simulink model "HW3_sim"  (R2024b)
settings: Solver=VariableStepAuto  StartTime=0.0  StopTime=sim_time  FixedStep=1  RelTol=1e-8  AbsTol=1e-8
values from neighbouring files (symbols this model uses):
  Ag0 = [sind(theta) 0 -sind(theta) 0; 0 sind(theta) 0 -sind(theta); cosd(theta) cosd(theta) cosd(theta) cosd(theta)]    [CMG_init_script.m]    (also in HW3_init_script.m)
  As0 = [sind(theta) 0 -sind(theta) 0; 0 sind(theta) 0 -sind(theta); cosd(theta) cosd(theta) cosd(theta) cosd(theta)]    [HW3_init_script.m]
  At0 = [-cosd(theta) 0 cosd(theta) 0; 0 -cosd(theta) 0 cosd(theta); sind(theta) sind(theta) sind(theta) sind(theta)]    [CMG_init_script.m]    (also in HW3_init_script.m)
  CMG = boolean(1)    [CMG_init_script.m]    (also in HW3_init_script.m)
  E0_body_ECI = euler_from_C(C0_body_ECI)    [CMG_init_script.m]    (also in HW3_init_script.m)
  E0_body_LVLH = euler_from_C(C0_body_LVLH)    [CMG_init_script.m]    (also in HW3_init_script.m)
  gamma0 = [0;0;0;0]    [CMG_init_script.m]    (also in HW3_init_script.m)
  I_b = 1/12*m_sc*diag([y^2 + z^2; x^2 + z^2; x^2 + y^2])    [CMG_init_script.m]    (also in HW3_init_script.m)
  I_cg = [I_CMG1(1,1) 0 0 0; 0 I_CMG2(1,1) 0 0; 0 0 I_CMG3(1,1) 0; 0 0 0 I_CMG4(1,1)]    [CMG_init_script.m]    (also in HW3_init_script.m)
  I_cs = I_ws    [CMG_init_script.m]    (also in HW3_init_script.m)
  I_ct = [I_CMG1(2,2) 0 0 0; 0 I_CMG2(2,2) 0 0; 0 0 I_CMG3(2,2) 0; 0 0 0 I_CMG4(2,2)]    [CMG_init_script.m]    (also in HW3_init_script.m)
  I_ws = [I_CMG1(3,3) 0 0 0; 0 I_CMG2(3,3) 0 0; 0 0 I_CMG3(3,3) 0; 0 0 0 I_CMG4(3,3)]    [CMG_init_script.m]    (also in HW3_init_script.m)
  J_sc = I_b + As0*I_cs*As0' + At0*I_ct*At0' + Ag0*I_cg*Ag0'    [CMG_init_script.m]    (also in HW3_init_script.m)
  K_d = 2*zeta*omega_n*J_sc    [CMG_init_script.m]    (also in HW3_init_script.m)
  K_p = 2*omega_n^2 * J_sc    [CMG_init_script.m]    (also in HW3_init_script.m)
  n_sc = (2*pi)/period    [CMG_init_script.m]    (also in HW3_init_script.m)
  Omega0 = [800; 800; 800; 800]    [CMG_init_script.m]    (also in HW3_init_script.m)
  omega0_body_ECI = 10^-3 * [0.5; -0.2; -3]    [CMG_init_script.m]    (also in HW3_init_script.m)
  q0_body_ECI = [0.5; 0.5; 0.5; 0.5]    [CMG_init_script.m]    (also in HW3_init_script.m)
  q0_body_LVLH = C2quat(C0_body_LVLH)    [CMG_init_script.m]    (also in HW3_init_script.m)
  q_c = [0; 0; 0; 1]    [CMG_init_script.m]    (also in HW3_init_script.m)
  r0 = r0'    [CMG_init_script.m]    (also in HW3_init_script.m)
  RW = boolean(0)    [CMG_init_script.m]    (also in HW3_init_script.m)
  T_d0 = 10^-5 * [0; 0.5; 0]    [CMG_init_script.m]    (also in HW3_init_script.m)
  v0 = v0'    [CMG_init_script.m]    (also in HW3_init_script.m)
settings Model: Creator=josep  LastModifiedBy=josep
settings DataIOCC: SaveFormat=StructureWithTime

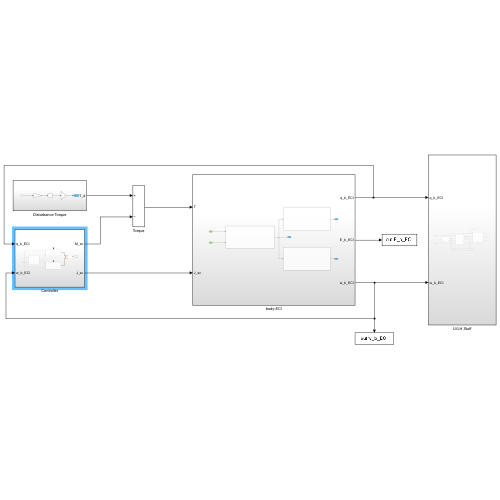
[thumbnail: Simulink's stored preview of the top-level diagram]
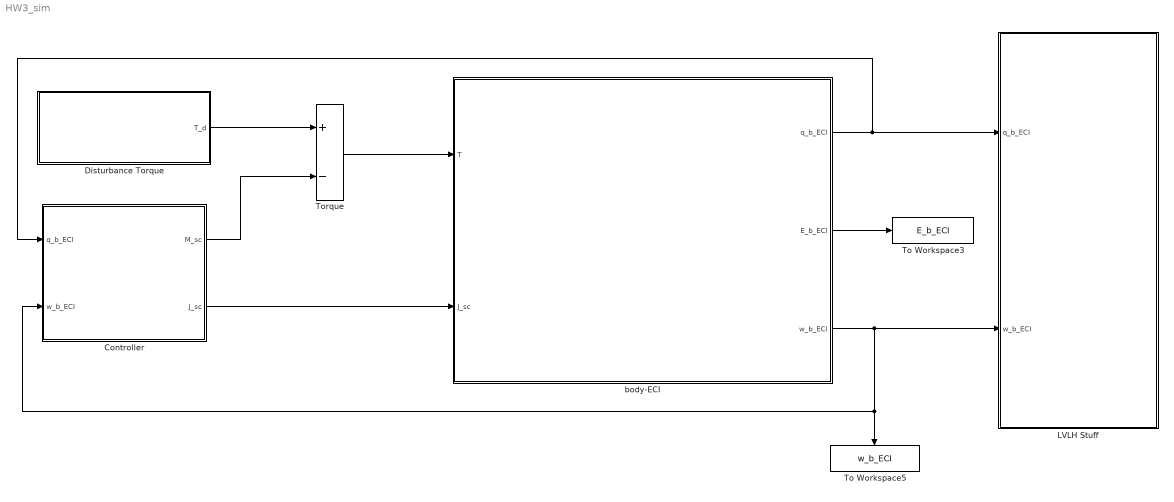
== system HW3_sim ==
  Controller : Subsystem
  Disturbance Torque : Subsystem
  LVLH Stuff : Subsystem
  To Workspace3 : ToWorkspace  VariableName=E_b_ECI  SampleTime=-1
  To Workspace5 : ToWorkspace  VariableName=w_b_ECI  SampleTime=-1
  Torque : Sum  Inputs=+-
  body-ECI : Subsystem
  wires:
  body-ECI/3(w_b_ECI) -> To Workspace5/1, Controller/2(w_b_ECI), LVLH Stuff/2(w_b_ECI)
  body-ECI/2(E_b_ECI) -> To Workspace3/1
  Torque/1 -> body-ECI/1(T)
  body-ECI/1(q_b_ECI) -> Controller/1(q_b_ECI), LVLH Stuff/1(q_b_ECI)
  Disturbance Torque/1(T_d) -> Torque/1
  Controller/2(J_sc) -> body-ECI/2(J_sc)
  Controller/1(M_sc) -> Torque/2

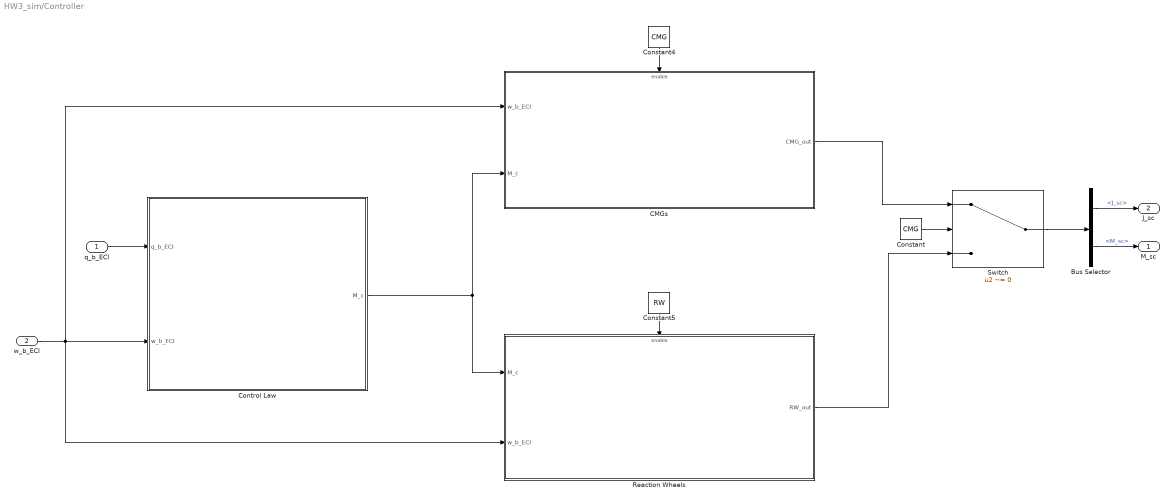
== system HW3_sim/Controller ==
  q_b_ECI : Inport
  w_b_ECI : Inport  Port=2
  Bus Selector : BusSelector  OutputSignals=J_sc,M_sc
  CMGs : Subsystem
  Constant : Constant  Value=CMG
  Constant4 : Constant  Value=CMG
  Constant5 : Constant  Value=RW
  Control Law : Subsystem
  Reaction Wheels : Subsystem
  Switch : Switch  Criteria=u2 ~= 0  SaturateOnIntegerOverflow=off  InputSameDT=off
  M_sc : Outport
  J_sc : Outport  Port=2
  wires:
  w_b_ECI/1 -> Reaction Wheels/2(w_b_ECI), CMGs/1(w_b_ECI), Control Law/2(w_b_ECI)
  Constant/1 -> Switch/2
  Constant4/1 -> CMGs/Enable
  Constant5/1 -> Reaction Wheels/Enable
  Switch/1 -> Bus Selector/1
  Bus Selector/1 -> J_sc/1  "<J_sc>"
  Bus Selector/2 -> M_sc/1  "<M_sc>"
  Control Law/1(M_c) -> CMGs/2(M_c), Reaction Wheels/1(M_c)
  q_b_ECI/1 -> Control Law/1(q_b_ECI)
  CMGs/1(CMG_out) -> Switch/1
  Reaction Wheels/1(RW_out) -> Switch/3

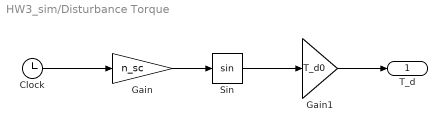
== system HW3_sim/Disturbance Torque ==
  Clock : Clock
  Gain : Gain  Gain=n_sc
  Gain1 : Gain  Gain=T_d0
  Sin : Trigonometry
  T_d : Outport
  wires:
  Gain1/1 -> T_d/1
  Clock/1 -> Gain/1
  Gain/1 -> Sin/1
  Sin/1 -> Gain1/1

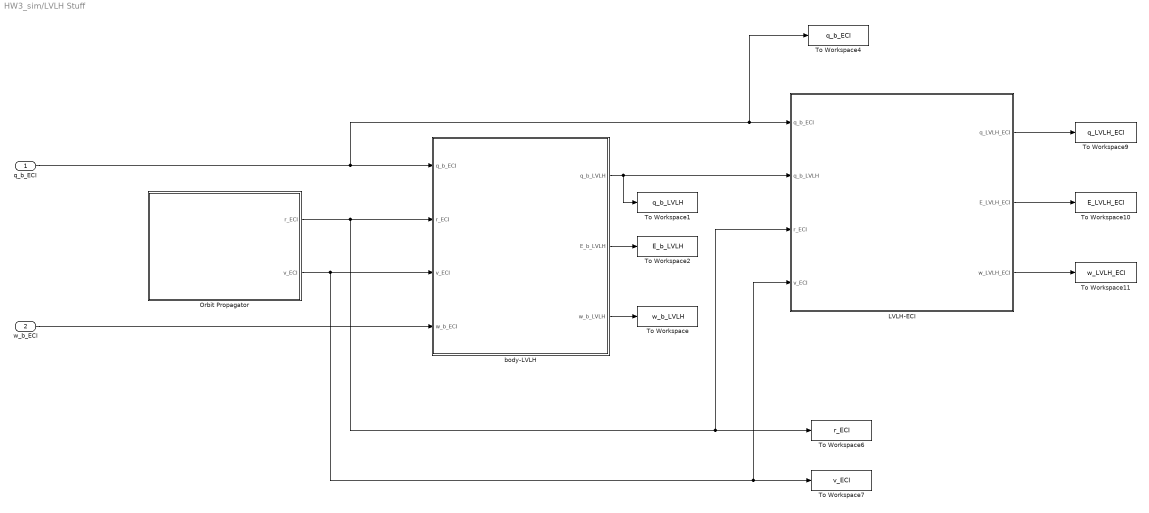
== system HW3_sim/LVLH Stuff ==
  q_b_ECI : Inport
  w_b_ECI : Inport  Port=2
  LVLH-ECI : Subsystem
  Orbit Propagator : Subsystem
  To Workspace : ToWorkspace  VariableName=w_b_LVLH  SampleTime=-1
  To Workspace1 : ToWorkspace  VariableName=q_b_LVLH  SampleTime=-1
      settings: Save2DSignal=2-D array (concatenate along first dimension)
  To Workspace10 : ToWorkspace  VariableName=E_LVLH_ECI  SampleTime=-1
  To Workspace11 : ToWorkspace  VariableName=w_LVLH_ECI  SampleTime=-1
  To Workspace2 : ToWorkspace  VariableName=E_b_LVLH  SampleTime=-1
  To Workspace4 : ToWorkspace  VariableName=q_b_ECI  SampleTime=-1
  To Workspace6 : ToWorkspace  VariableName=r_ECI  SampleTime=-1
  To Workspace7 : ToWorkspace  VariableName=v_ECI  SampleTime=-1
  To Workspace9 : ToWorkspace  VariableName=q_LVLH_ECI  SampleTime=-1
  body-LVLH : Subsystem
  wires:
  q_b_ECI/1 -> LVLH-ECI/1(q_b_ECI), To Workspace4/1, body-LVLH/1(q_b_ECI)
  body-LVLH/3(w_b_LVLH) -> To Workspace/1
  Orbit Propagator/2(v_ECI) -> body-LVLH/3(v_ECI), LVLH-ECI/4(v_ECI), To Workspace7/1
  body-LVLH/2(E_b_LVLH) -> To Workspace2/1
  LVLH-ECI/1(q_LVLH_ECI) -> To Workspace9/1
  Orbit Propagator/1(r_ECI) -> body-LVLH/2(r_ECI), To Workspace6/1, LVLH-ECI/3(r_ECI)
  LVLH-ECI/3(w_LVLH_ECI) -> To Workspace11/1
  body-LVLH/1(q_b_LVLH) -> LVLH-ECI/2(q_b_LVLH), To Workspace1/1
  LVLH-ECI/2(E_LVLH_ECI) -> To Workspace10/1
  w_b_ECI/1 -> body-LVLH/4(w_b_ECI)

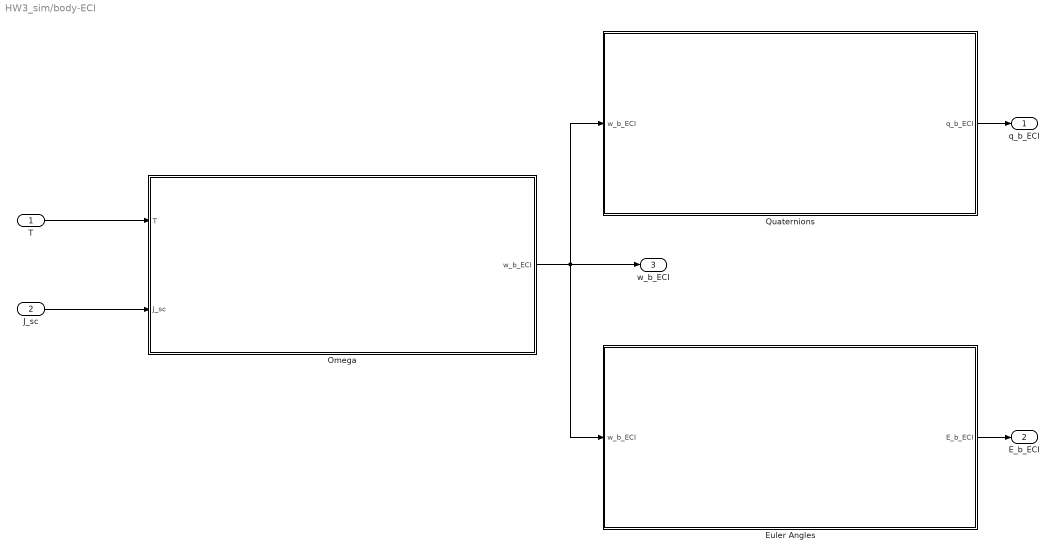
== system HW3_sim/body-ECI ==
  T : Inport
  J_sc : Inport  Port=2
  Euler Angles : Subsystem
  Omega : Subsystem
  Quaternions : Subsystem
  q_b_ECI : Outport
  E_b_ECI : Outport  Port=2
  w_b_ECI : Outport  Port=3
  wires:
  Omega/1(w_b_ECI) -> Quaternions/1(w_b_ECI), Euler Angles/1(w_b_ECI), w_b_ECI/1
  Euler Angles/1(E_b_ECI) -> E_b_ECI/1
  Quaternions/1(q_b_ECI) -> q_b_ECI/1
  T/1 -> Omega/1(T)
  J_sc/1 -> Omega/2(J_sc)

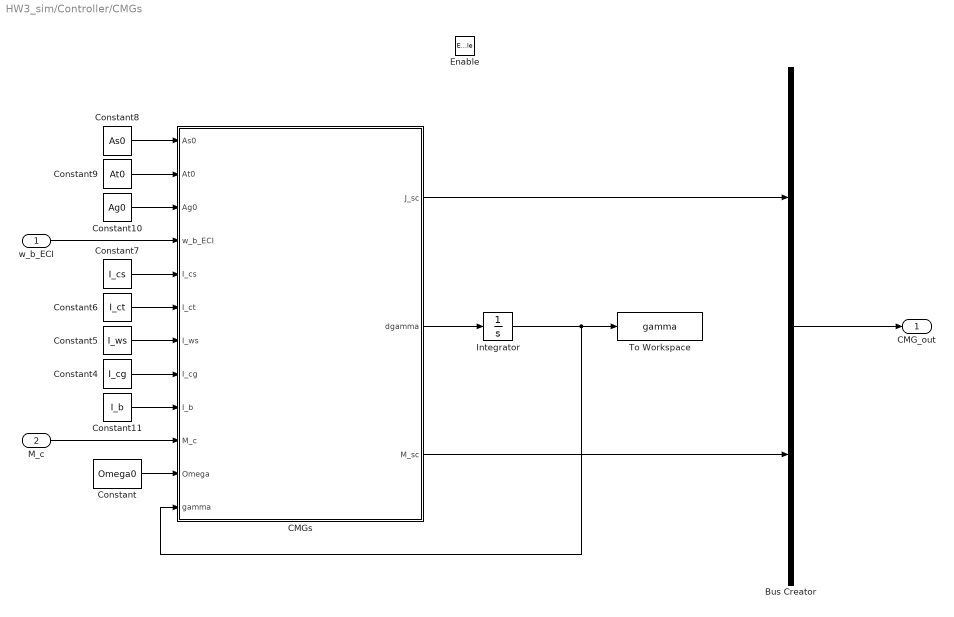
== system HW3_sim/Controller/CMGs ==
  w_b_ECI : Inport
  M_c : Inport  Port=2
  Enable : EnablePort
  Bus Creator : BusCreator  Inputs=2
  CMGs : MATLAB Function  TreatAsAtomicUnit=on
  Constant : Constant  Value=Omega0
  Constant10 : Constant  Value=Ag0
  Constant11 : Constant  Value=I_b
  Constant4 : Constant  Value=I_cg
  Constant5 : Constant  Value=I_ws
  Constant6 : Constant  Value=I_ct
  Constant7 : Constant  Value=I_cs
  Constant8 : Constant  Value=As0
  Constant9 : Constant  Value=At0
  Integrator : Integrator  InitialCondition=gamma0
  To Workspace : ToWorkspace  VariableName=gamma  SampleTime=-1
  CMG_out : Outport
  wires:
  Constant5/1 -> CMGs/7(I_ws)
  Constant4/1 -> CMGs/8(I_cg)
  Constant11/1 -> CMGs/9(I_b)
  Constant10/1 -> CMGs/3(Ag0)
  Constant7/1 -> CMGs/5(I_cs)
  Constant/1 -> CMGs/11(Omega)
  Integrator/1 -> To Workspace/1, CMGs/12(gamma)
  Constant6/1 -> CMGs/6(I_ct)
  Constant9/1 -> CMGs/2(At0)
  CMGs/2(dgamma) -> Integrator/1
  Constant8/1 -> CMGs/1(As0)
  M_c/1 -> CMGs/10(M_c)
  w_b_ECI/1 -> CMGs/4(w_b_ECI)
  CMGs/1(J_sc) -> Bus Creator/1
  CMGs/3(M_sc) -> Bus Creator/2
  Bus Creator/1 -> CMG_out/1

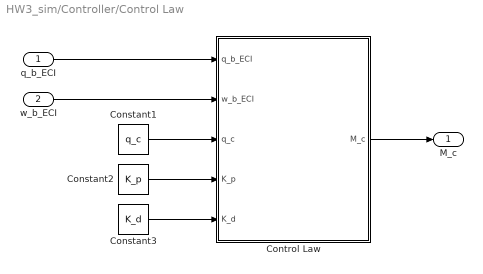
== system HW3_sim/Controller/Control Law ==
  q_b_ECI : Inport
  w_b_ECI : Inport  Port=2
  Constant1 : Constant  Value=q_c
  Constant2 : Constant  Value=K_p
  Constant3 : Constant  Value=K_d
  Control Law : MATLAB Function  TreatAsAtomicUnit=on
  M_c : Outport
  wires:
  Constant1/1 -> Control Law/3(q_c)
  Constant3/1 -> Control Law/5(K_d)
  Constant2/1 -> Control Law/4(K_p)
  q_b_ECI/1 -> Control Law/1(q_b_ECI)
  Control Law/1(M_c) -> M_c/1
  w_b_ECI/1 -> Control Law/2(w_b_ECI)

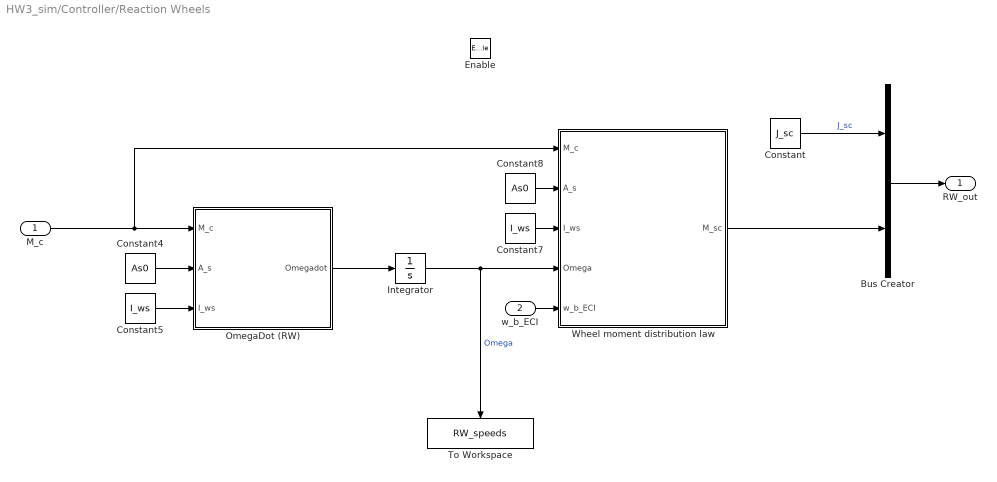
== system HW3_sim/Controller/Reaction Wheels ==
  M_c : Inport
  w_b_ECI : Inport  Port=2
  Enable : EnablePort
  Bus Creator : BusCreator  Inputs=2
  Constant : Constant  Value=J_sc
  Constant4 : Constant  Value=As0
  Constant5 : Constant  Value=I_ws
  Constant7 : Constant  Value=I_ws
  Constant8 : Constant  Value=As0
  Integrator : Integrator  InitialCondition=Omega0
  OmegaDot (RW) : MATLAB Function  TreatAsAtomicUnit=on
  To Workspace : ToWorkspace  VariableName=RW_speeds  SampleTime=-1
  Wheel moment distribution law : MATLAB Function  TreatAsAtomicUnit=on
  RW_out : Outport
  wires:
  Constant5/1 -> OmegaDot (RW)/3(I_ws)
  Integrator/1 -> Wheel moment distribution law/4(Omega), To Workspace/1  "Omega"
  Constant4/1 -> OmegaDot (RW)/2(A_s)
  OmegaDot (RW)/1(Omegadot) -> Integrator/1
  Constant8/1 -> Wheel moment distribution law/2(A_s)
  Constant7/1 -> Wheel moment distribution law/3(I_ws)
  w_b_ECI/1 -> Wheel moment distribution law/5(w_b_ECI)
  M_c/1 -> Wheel moment distribution law/1(M_c), OmegaDot (RW)/1(M_c)
  Bus Creator/1 -> RW_out/1
  Constant/1 -> Bus Creator/1  "J_sc"
  Wheel moment distribution law/1(M_sc) -> Bus Creator/2

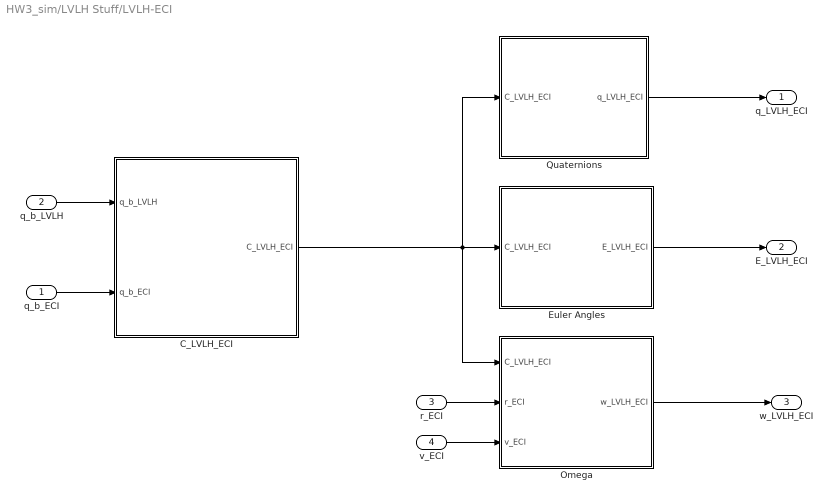
== system HW3_sim/LVLH Stuff/LVLH-ECI ==
  q_b_ECI : Inport
  q_b_LVLH : Inport  Port=2
  r_ECI : Inport  Port=3
  v_ECI : Inport  Port=4
  C_LVLH_ECI : MATLAB Function  TreatAsAtomicUnit=on
  Euler Angles : MATLAB Function  TreatAsAtomicUnit=on
  Omega : MATLAB Function  TreatAsAtomicUnit=on
  Quaternions : MATLAB Function  TreatAsAtomicUnit=on
  q_LVLH_ECI : Outport
  E_LVLH_ECI : Outport  Port=2
  w_LVLH_ECI : Outport  Port=3
  wires:
  q_b_LVLH/1 -> C_LVLH_ECI/1(q_b_LVLH)
  q_b_ECI/1 -> C_LVLH_ECI/2(q_b_ECI)
  C_LVLH_ECI/1(C_LVLH_ECI) -> Quaternions/1(C_LVLH_ECI), Omega/1(C_LVLH_ECI), Euler Angles/1(C_LVLH_ECI)
  r_ECI/1 -> Omega/2(r_ECI)
  v_ECI/1 -> Omega/3(v_ECI)
  Quaternions/1(q_LVLH_ECI) -> q_LVLH_ECI/1
  Euler Angles/1(E_LVLH_ECI) -> E_LVLH_ECI/1
  Omega/1(w_LVLH_ECI) -> w_LVLH_ECI/1

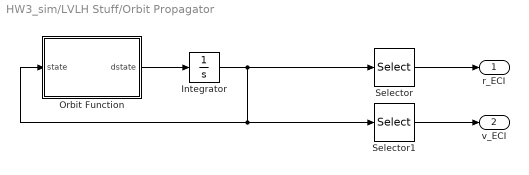
== system HW3_sim/LVLH Stuff/Orbit Propagator ==
  Integrator : Integrator  InitialCondition=[r0; v0]
  Orbit Function : MATLAB Function  TreatAsAtomicUnit=on
  Selector : Selector  InputPortWidth=6  IndexOptions=Index vector (dialog)  Indices=[1; 2; 3]  OutputSizes=1
  Selector1 : Selector  InputPortWidth=6  IndexOptions=Index vector (dialog)  Indices=[4; 5; 6]  OutputSizes=1
  r_ECI : Outport
  v_ECI : Outport  Port=2
  wires:
  Integrator/1 -> Orbit Function/1(state), Selector1/1, Selector/1
  Orbit Function/1(dstate) -> Integrator/1
  Selector/1 -> r_ECI/1
  Selector1/1 -> v_ECI/1

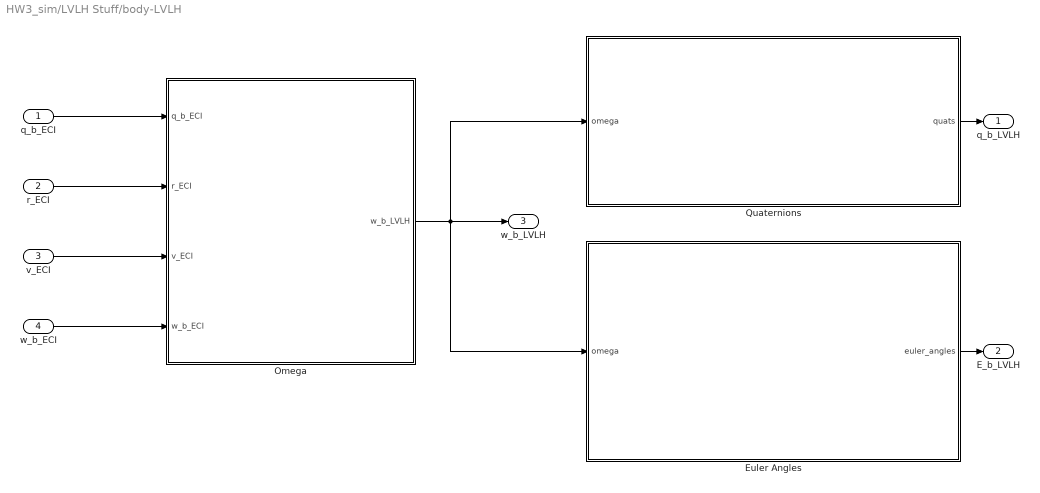
== system HW3_sim/LVLH Stuff/body-LVLH ==
  q_b_ECI : Inport
  r_ECI : Inport  Port=2
  v_ECI : Inport  Port=3
  w_b_ECI : Inport  Port=4
  Euler Angles : Subsystem
  Omega : Subsystem
  Quaternions : Subsystem
  q_b_LVLH : Outport
  E_b_LVLH : Outport  Port=2
  w_b_LVLH : Outport  Port=3
  wires:
  Omega/1(w_b_LVLH) -> Quaternions/1(omega), Euler Angles/1(omega), w_b_LVLH/1
  q_b_ECI/1 -> Omega/1(q_b_ECI)
  r_ECI/1 -> Omega/2(r_ECI)
  v_ECI/1 -> Omega/3(v_ECI)
  w_b_ECI/1 -> Omega/4(w_b_ECI)
  Euler Angles/1(euler_angles) -> E_b_LVLH/1
  Quaternions/1(quats) -> q_b_LVLH/1

== system HW3_sim/body-ECI/Euler Angles ==
  w_b_ECI : Inport
  Integrator1 : Integrator  InitialCondition=E0_body_ECI
  dEuler : MATLAB Function  TreatAsAtomicUnit=on
  E_b_ECI : Outport
  wires:
  Integrator1/1 -> E_b_ECI/1, dEuler/2(euler_angles)
  dEuler/1(dEuler) -> Integrator1/1
  w_b_ECI/1 -> dEuler/1(omega)

== system HW3_sim/body-ECI/Omega ==
  T : Inport
  J_sc : Inport  Port=2
  Integrator : Integrator  InitialCondition=omega0_body_ECI
  domega : MATLAB Function  TreatAsAtomicUnit=on
  w_b_ECI : Outport
  wires:
  T/1 -> domega/1(T)
  domega/1(domega) -> Integrator/1
  Integrator/1 -> w_b_ECI/1, domega/3(omega)
  J_sc/1 -> domega/2(J)

== system HW3_sim/body-ECI/Quaternions ==
  w_b_ECI : Inport
  Integrator2 : Integrator  InitialCondition=q0_body_ECI
  dQuats : MATLAB Function  TreatAsAtomicUnit=on
  q_b_ECI : Outport
  wires:
  w_b_ECI/1 -> dQuats/1(omega)
  dQuats/1(dquats) -> Integrator2/1
  Integrator2/1 -> q_b_ECI/1, dQuats/2(quats)

== system HW3_sim/LVLH Stuff/body-LVLH/Euler Angles ==
  omega : Inport
  Integrator : Integrator  InitialCondition=E0_body_LVLH
  dEuler : MATLAB Function  TreatAsAtomicUnit=on
  euler_angles : Outport
  wires:
  Integrator/1 -> euler_angles/1, dEuler/2(euler_angles)
  dEuler/1(dEuler) -> Integrator/1
  omega/1 -> dEuler/1(omega)

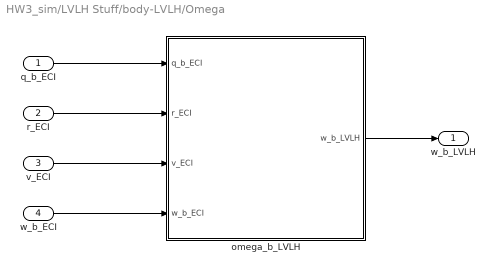
== system HW3_sim/LVLH Stuff/body-LVLH/Omega ==
  q_b_ECI : Inport
  r_ECI : Inport  Port=2
  v_ECI : Inport  Port=3
  w_b_ECI : Inport  Port=4
  omega_b_LVLH : MATLAB Function  TreatAsAtomicUnit=on
  w_b_LVLH : Outport
  wires:
  r_ECI/1 -> omega_b_LVLH/2(r_ECI)
  q_b_ECI/1 -> omega_b_LVLH/1(q_b_ECI)
  w_b_ECI/1 -> omega_b_LVLH/4(w_b_ECI)
  v_ECI/1 -> omega_b_LVLH/3(v_ECI)
  omega_b_LVLH/1(w_b_LVLH) -> w_b_LVLH/1

== system HW3_sim/LVLH Stuff/body-LVLH/Quaternions ==
  omega : Inport
  Integrator2 : Integrator  InitialCondition=q0_body_LVLH
  dQuats : MATLAB Function  TreatAsAtomicUnit=on
  quats : Outport
  wires:
  Integrator2/1 -> quats/1, dQuats/2(quats)
  dQuats/1(dquats) -> Integrator2/1
  omega/1 -> dQuats/1(omega)

== matlab function HW3_sim/LVLH Stuff/LVLH-ECI/Euler Angles ==
  data: C_LVLH_ECI input; E_LVLH_ECI output
function E_LVLH_ECI = fcn(C_LVLH_ECI)

E_LVLH_ECI = euler_from_C(C_LVLH_ECI);

== matlab function HW3_sim/LVLH Stuff/LVLH-ECI/Omega ==
  data: C_LVLH_ECI input; w_LVLH_ECI output; r_ECI input; v_ECI input
function w_LVLH_ECI = fcn(C_LVLH_ECI, r_ECI, v_ECI)

w_LVLH_ECI = C_LVLH_ECI * (cross(r_ECI, v_ECI) / norm(r_ECI)^2);

== matlab function HW3_sim/Controller/CMGs/CMGs ==
  data: J_sc output; As0 input; dgamma output; At0 input; Ag0 input; w_b_ECI input; I_cs input; I_ct input; I_ws input; I_cg input; I_b input; M_c input; Omega input; gamma input; M_sc output
function [J_sc, dgamma, M_sc] = fcn(As0, At0, Ag0, w_b_ECI, I_cs, I_ct, I_ws, I_cg, I_b, M_c, Omega, gamma)

A_s = (As0 * diag(cos(gamma))) + (At0*(diag(sin(gamma))));
A_t = (At0 * diag(cos(gamma))) - (As0*(diag(sin(gamma))));
A_g = Ag0;

J_sc = I_b + A_s*I_cs*A_s' + A_t*I_ct*A_t' + A_g*I_cg*A_g';

N = 4;
C1 = zeros(3,N); C2 = C1;
for i = 1:N
    C1(:,i) = A_t(:,i)*A_s(:,i)'*w_b_ECI;
    C2(:,i) = A_s(:,i)*A_t(:,i)'*w_b_ECI;
end
C = C1+C2;

Q = (A_t*I_ws*diag(Omega)) + vect2cross(w_b_ECI)*(A_g*I_cg) + C*(I_cs-I_ct);
% alpha = exp(-det(Q*Q'));

dgamma = pinv(Q)*M_c;


M_sc = M_c + vect2cross(w_b_ECI)*A_s*I_ws*Omega;

== matlab function HW3_sim/Controller/Reaction Wheels/OmegaDot (RW) ==
  data: M_c input; Omegadot output; A_s input; I_ws input
function Omegadot = fcn(M_c, A_s, I_ws)

Omegadot = (I_ws) \ pinv(A_s) * M_c;

== matlab function HW3_sim/Controller/Reaction Wheels/Wheel moment distribution law ==
  data: M_c input; M_sc output; A_s input; I_ws input; Omega input; w_b_ECI input
function M_sc = fcn(M_c, A_s, I_ws, Omega, w_b_ECI)

M_sc =  M_c + (cross(w_b_ECI, (A_s *I_ws* Omega)));

== matlab function HW3_sim/Controller/Control Law/Control Law ==
  data: M_c output; q_b_ECI input; w_b_ECI input; q_c input; K_p input; K_d input
function M_c   = fcn(q_b_ECI, w_b_ECI, q_c, K_p, K_d)

q_e = quatmult(q_b_ECI, quatconjugate(q_c));

eta_e = q_e(4);
eps_e = q_e(1:3);

M_c = K_p*eps_e*sign(eta_e) + (K_d*w_b_ECI);

== matlab function HW3_sim/body-ECI/Omega/domega ==
  data: T input; domega output; J input; omega input
function domega = fcn(T, J, omega)



domega = J\(T - cross(omega, (J*omega)));

== matlab function HW3_sim/LVLH Stuff/LVLH-ECI/C_LVLH_ECI ==
  data: q_b_LVLH input; C_LVLH_ECI output; q_b_ECI input
function C_LVLH_ECI = fcn(q_b_LVLH, q_b_ECI)

C_b_LVLH = quat2C(q_b_LVLH);
C_LVLH_b = C_b_LVLH';

C_b_ECI = quat2C(q_b_ECI);

C_LVLH_ECI = C_LVLH_b*C_b_ECI;

== matlab function HW3_sim/LVLH Stuff/Orbit Propagator/Orbit Function ==
  data: state input; dstate output
function dstate = two_body(state)

mu = 398600.4418;

x = state(1);
y = state(2);
z = state(3);

dx = state(4);
dy = state(5);
dz = state(6);

r = norm([x y z]);

ddx = -mu*x/r^3;
ddy = -mu*y/r^3;
ddz = -mu*z/r^3;


dstate = [dx; dy; dz; ddx; ddy; ddz];
end

== matlab function HW3_sim/LVLH Stuff/LVLH-ECI/Quaternions ==
  data: C_LVLH_ECI input; q_LVLH_ECI output
function q_LVLH_ECI = fcn(C_LVLH_ECI)

q_LVLH_ECI = C2quat(C_LVLH_ECI);

== matlab function HW3_sim/body-ECI/Euler Angles/dEuler ==
  data: omega input; dEuler output; euler_angles input
function dEuler = fcn(omega, euler_angles)

dEuler = [1 sin(euler_angles(1))*tan(euler_angles(2)) cos(euler_angles(1))*tan(euler_angles(2));...
            0 cos(euler_angles(1)) -sin(euler_angles(1));...
            0 sin(euler_angles(1))*sec(euler_angles(2)) cos(euler_angles(1))*sec(euler_angles(2))] * omega;

== matlab function HW3_sim/LVLH Stuff/body-LVLH/Euler Angles/dEuler ==
  data: omega input; dEuler output; euler_angles input
function dEuler = fcn(omega, euler_angles)

dEuler = [1 sin(euler_angles(1))*tan(euler_angles(2)) cos(euler_angles(1))*tan(euler_angles(2));...
            0 cos(euler_angles(1)) -sin(euler_angles(1));...
            0 sin(euler_angles(1))*sec(euler_angles(2)) cos(euler_angles(1))*sec(euler_angles(2))] * omega;

== matlab function HW3_sim/LVLH Stuff/body-LVLH/Omega/omega_b_LVLH ==
  data: q_b_ECI input; w_b_LVLH output; r_ECI input; v_ECI input; w_b_ECI input
function w_b_LVLH   = fcn(q_b_ECI, r_ECI, v_ECI, w_b_ECI)

C_b_ECI = quat2C(q_b_ECI);

w_LVLH_ECI = cross(r_ECI, v_ECI)/norm(r_ECI)^2;

w_b_LVLH = w_b_ECI - (C_b_ECI*w_LVLH_ECI);


end

== matlab function HW3_sim/LVLH Stuff/body-LVLH/Quaternions/dQuats ==
  data: omega input; dquats output; quats input
function dquats = fcn(omega, quats)

eta = quats(4);
eps = quats(1:3);
eps_dot = 0.5*(eta*eye(3) + vect2cross(eps))*omega;
eta_dot = -0.5*eps'*omega;

dquats = [eps_dot; eta_dot];

== matlab function HW3_sim/body-ECI/Quaternions/dQuats ==
  data: omega input; dquats output; quats input
function dquats = fcn(omega, quats)

eta = quats(4);
eps = quats(1:3);
eps_dot = 0.5*(eta*eye(3) + vect2cross(eps))*omega;
eta_dot = -0.5*eps'*omega;

dquats = [eps_dot; eta_dot];
